simulink model "sumulink_stepping"  (R2017a)
settings: Solver=VariableStepAuto  StartTime=0.0  StopTime=10.0  RelTol=1e-3
settings Model: Creator=lenovo  LastModifiedBy=lenovo
settings DataIOCC: SaveFormat=Array

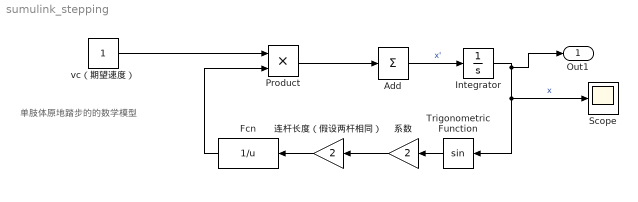
== system sumulink_stepping ==
  note: 单肢体原地踏步的的数学模型
  Add : Sum  Inputs=+
  Fcn : Fcn  Expr=1/u
  Integrator : Integrator  InitialCondition=0.1
  Product : Product
  Scope : Scope
  Trigonometric Function : Trigonometry
  vc（期望速度） : Constant
  系数 : Gain  Gain=2
  连杆长度（假设两杆相同） : Gain  Gain=2
  Out1 : Outport
  wires:
  Add/1 -> Integrator/1  "x'"
  Integrator/1 -> Out1/1, Scope/1, Trigonometric Function/1  "x"
  Trigonometric Function/1 -> 系数/1
  系数/1 -> 连杆长度（假设两杆相同）/1
  连杆长度（假设两杆相同）/1 -> Fcn/1
  Product/1 -> Add/1
  Fcn/1 -> Product/2
  vc（期望速度）/1 -> Product/1
